simulink model "Microwave"  (Simulink 8.7)
settings: Solver=ode45  StartTime=0.0  StopTime=20  RelTol=1e-3
libraries: simulink x16
settings Model: Creator=bourbouh  LastModifiedBy=bourbouh
settings DataIOCC: SaveFormat=Structure
settings DebuggingCC: UnderspecifiedInitializationDetection=Simplified  MergeDetectMultiDrivingBlocksExec=error

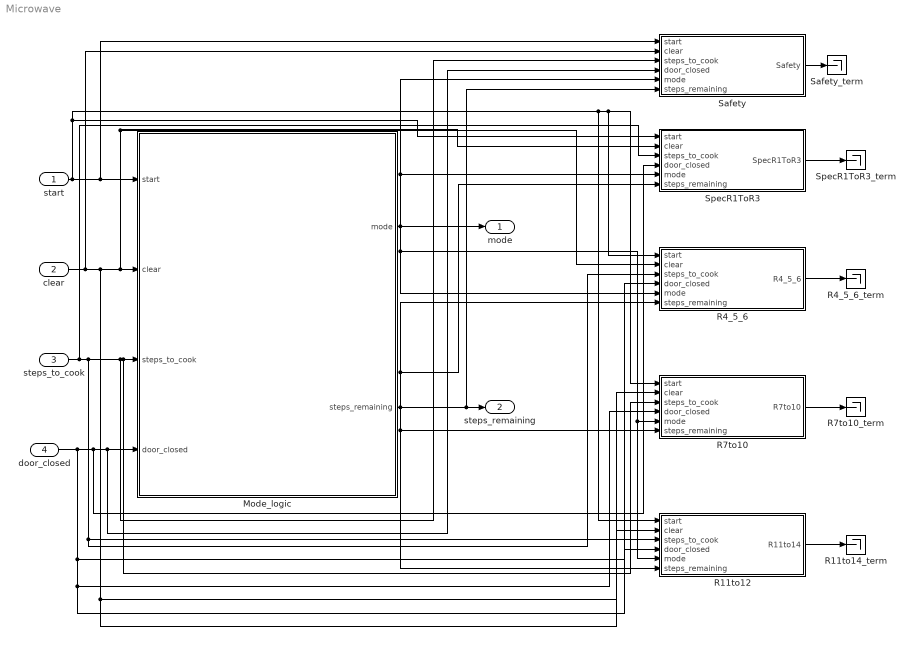
== system Microwave ==
  start : Inport
  clear : Inport  Port=2
  steps_to_cook : Inport  Port=3
  door_closed : Inport  Port=4
  Mode_logic : Stateflow chart  TreatAsAtomicUnit=on
  R11to12 : Subsystem  TreatAsAtomicUnit=on  mask(Observer){AnnotationType=ensures, ObserverType=[]}
      mask prompts: AnnotationType "Type of annotation (pre/post...)"; ObserverType "Observer type"
      mask help:
      | Set an observer for the system.
      | The annotation type parameter sets the type of observer:
      | - requires : pre-condition
      | - ensures : post-condition
      | - assert : an assertion
      | - observer : the observer computes a special type of properties
      mask TypeOptions AnnotationType: ensures | requires | assert | observer
      mask Callback AnnotationType:
      | paramStr = get_param(gcb, 'MaskValues');
      | if strcmp(paramStr{1}(1),'o')
      | set_param(gcb,'MaskVisibilities',{'on';'on'});
      | paramStr{2} = 'ellipsoid';
      | set_param(gcb,'MaskValues',paramStr);
      | else
      | set_param(gcb,'MaskVisibilities',{'on';'off'});
      | end
      | clear paramStr;
      mask Callback ObserverType:
      | paramStr = get_param(gcb, 'MaskValues');
      | if strcmp(paramStr{1}(1),'o')
      | set_param(gcb,'MaskVisibilities',{'on';'on'});
      | paramStr{2} = 'ellipsoid';
      | set_param(gcb,'MaskValues',paramStr);
      | else
      | set_param(gcb,'MaskVisibilities',{'on';'off'});
      | end
      | clear paramStr;
      mask Display:
      | color('black')
      | text(0.5, 0.5, ['Property: ''' get_param(gcb,'name') ''''], 'horizontalAlignment', 'center');
      | text(0.99, 0.03, '{\bf\fontsize{12}SAFE}', 'hor', 'right', 'ver', 'bottom', 'texmode', 'on');
  R11to14_term : Terminator
  R4_5_6 : Subsystem  TreatAsAtomicUnit=on  mask(Observer){AnnotationType=ensures, ObserverType=[]}
      mask prompts: AnnotationType "Type of annotation (pre/post...)"; ObserverType "Observer type"
      mask help:
      | Set an observer for the system.
      | The annotation type parameter sets the type of observer:
      | - requires : pre-condition
      | - ensures : post-condition
      | - assert : an assertion
      | - observer : the observer computes a special type of properties
      mask TypeOptions AnnotationType: ensures | requires | assert | observer
      mask Callback AnnotationType:
      | paramStr = get_param(gcb, 'MaskValues');
      | if strcmp(paramStr{1}(1),'o')
      | set_param(gcb,'MaskVisibilities',{'on';'on'});
      | paramStr{2} = 'ellipsoid';
      | set_param(gcb,'MaskValues',paramStr);
      | else
      | set_param(gcb,'MaskVisibilities',{'on';'off'});
      | end
      | clear paramStr;
      mask Callback ObserverType:
      | paramStr = get_param(gcb, 'MaskValues');
      | if strcmp(paramStr{1}(1),'o')
      | set_param(gcb,'MaskVisibilities',{'on';'on'});
      | paramStr{2} = 'ellipsoid';
      | set_param(gcb,'MaskValues',paramStr);
      | else
      | set_param(gcb,'MaskVisibilities',{'on';'off'});
      | end
      | clear paramStr;
      mask Display:
      | color('black')
      | text(0.5, 0.5, ['Property: ''' get_param(gcb,'name') ''''], 'horizontalAlignment', 'center');
      | text(0.99, 0.03, '{\bf\fontsize{12}SAFE}', 'hor', 'right', 'ver', 'bottom', 'texmode', 'on');
  R4_5_6_term : Terminator
  R7to10 : Subsystem  TreatAsAtomicUnit=on  mask(Observer){AnnotationType=ensures, ObserverType=[]}
      mask prompts: AnnotationType "Type of annotation (pre/post...)"; ObserverType "Observer type"
      mask help:
      | Set an observer for the system.
      | The annotation type parameter sets the type of observer:
      | - requires : pre-condition
      | - ensures : post-condition
      | - assert : an assertion
      | - observer : the observer computes a special type of properties
      mask TypeOptions AnnotationType: ensures | requires | assert | observer
      mask Callback AnnotationType:
      | paramStr = get_param(gcb, 'MaskValues');
      | if strcmp(paramStr{1}(1),'o')
      | set_param(gcb,'MaskVisibilities',{'on';'on'});
      | paramStr{2} = 'ellipsoid';
      | set_param(gcb,'MaskValues',paramStr);
      | else
      | set_param(gcb,'MaskVisibilities',{'on';'off'});
      | end
      | clear paramStr;
      mask Callback ObserverType:
      | paramStr = get_param(gcb, 'MaskValues');
      | if strcmp(paramStr{1}(1),'o')
      | set_param(gcb,'MaskVisibilities',{'on';'on'});
      | paramStr{2} = 'ellipsoid';
      | set_param(gcb,'MaskValues',paramStr);
      | else
      | set_param(gcb,'MaskVisibilities',{'on';'off'});
      | end
      | clear paramStr;
      mask Display:
      | color('black')
      | text(0.5, 0.5, ['Property: ''' get_param(gcb,'name') ''''], 'horizontalAlignment', 'center');
      | text(0.99, 0.03, '{\bf\fontsize{12}SAFE}', 'hor', 'right', 'ver', 'bottom', 'texmode', 'on');
  R7to10_term : Terminator
  Safety : Subsystem  TreatAsAtomicUnit=on  mask(Observer){AnnotationType=ensures, ObserverType=[]}
      mask prompts: AnnotationType "Type of annotation (pre/post...)"; ObserverType "Observer type"
      mask help:
      | Set an observer for the system.
      | The annotation type parameter sets the type of observer:
      | - requires : pre-condition
      | - ensures : post-condition
      | - assert : an assertion
      | - observer : the observer computes a special type of properties
      mask TypeOptions AnnotationType: ensures | requires | assert | observer
      mask Callback AnnotationType:
      | paramStr = get_param(gcb, 'MaskValues');
      | if strcmp(paramStr{1}(1),'o')
      | set_param(gcb,'MaskVisibilities',{'on';'on'});
      | paramStr{2} = 'ellipsoid';
      | set_param(gcb,'MaskValues',paramStr);
      | else
      | set_param(gcb,'MaskVisibilities',{'on';'off'});
      | end
      | clear paramStr;
      mask Callback ObserverType:
      | paramStr = get_param(gcb, 'MaskValues');
      | if strcmp(paramStr{1}(1),'o')
      | set_param(gcb,'MaskVisibilities',{'on';'on'});
      | paramStr{2} = 'ellipsoid';
      | set_param(gcb,'MaskValues',paramStr);
      | else
      | set_param(gcb,'MaskVisibilities',{'on';'off'});
      | end
      | clear paramStr;
      mask Display:
      | color('black')
      | text(0.5, 0.5, ['Property: ''' get_param(gcb,'name') ''''], 'horizontalAlignment', 'center');
      | text(0.99, 0.03, '{\bf\fontsize{12}SAFE}', 'hor', 'right', 'ver', 'bottom', 'texmode', 'on');
  Safety_term : Terminator
  SpecR1ToR3 : Subsystem  TreatAsAtomicUnit=on  mask(Observer){AnnotationType=ensures, ObserverType=[]}
      mask prompts: AnnotationType "Type of annotation (pre/post...)"; ObserverType "Observer type"
      mask help:
      | Set an observer for the system.
      | The annotation type parameter sets the type of observer:
      | - requires : pre-condition
      | - ensures : post-condition
      | - assert : an assertion
      | - observer : the observer computes a special type of properties
      mask TypeOptions AnnotationType: ensures | requires | assert | observer
      mask Callback AnnotationType:
      | paramStr = get_param(gcb, 'MaskValues');
      | if strcmp(paramStr{1}(1),'o')
      | set_param(gcb,'MaskVisibilities',{'on';'on'});
      | paramStr{2} = 'ellipsoid';
      | set_param(gcb,'MaskValues',paramStr);
      | else
      | set_param(gcb,'MaskVisibilities',{'on';'off'});
      | end
      | clear paramStr;
      mask Callback ObserverType:
      | paramStr = get_param(gcb, 'MaskValues');
      | if strcmp(paramStr{1}(1),'o')
      | set_param(gcb,'MaskVisibilities',{'on';'on'});
      | paramStr{2} = 'ellipsoid';
      | set_param(gcb,'MaskValues',paramStr);
      | else
      | set_param(gcb,'MaskVisibilities',{'on';'off'});
      | end
      | clear paramStr;
      mask Display:
      | color('black')
      | text(0.5, 0.5, ['Property: ''' get_param(gcb,'name') ''''], 'horizontalAlignment', 'center');
      | text(0.99, 0.03, '{\bf\fontsize{12}SAFE}', 'hor', 'right', 'ver', 'bottom', 'texmode', 'on');
  SpecR1ToR3_term : Terminator
  mode : Outport
  steps_remaining : Outport  Port=2
  wires:
  start/1 -> R11to12/1(start), R7to10/1(start), R4_5_6/1(start), SpecR1ToR3/1(start), Safety/1(start), Mode_logic/1(start)
  door_closed/1 -> R11to12/4(door_closed), R7to10/4(door_closed), R4_5_6/4(door_closed), Mode_logic/4(door_closed), Safety/4(door_closed), SpecR1ToR3/4(door_closed)
  steps_to_cook/1 -> R11to12/3(steps_to_cook), R4_5_6/3(steps_to_cook), R7to10/3(steps_to_cook), Mode_logic/3(steps_to_cook), Safety/3(steps_to_cook), SpecR1ToR3/3(steps_to_cook)
  clear/1 -> R11to12/2(clear), R7to10/2(clear), R4_5_6/2(clear), SpecR1ToR3/2(clear), Mode_logic/2(clear), Safety/2(clear)
  Mode_logic/1(mode) -> R11to12/5(mode), R7to10/5(mode), R4_5_6/5(mode), Safety/5(mode), SpecR1ToR3/5(mode), mode/1
  Mode_logic/2(steps_remaining) -> R7to10/6(steps_remaining), R11to12/6(steps_remaining), SpecR1ToR3/6(steps_remaining), R4_5_6/6(steps_remaining), steps_remaining/1, Safety/6(steps_remaining)
  Safety/1(Safety) -> Safety_term/1
  SpecR1ToR3/1(SpecR1ToR3) -> SpecR1ToR3_term/1
  R4_5_6/1(R4_5_6) -> R4_5_6_term/1
  R7to10/1(R7to10) -> R7to10_term/1
  R11to12/1(R11to14) -> R11to14_term/1

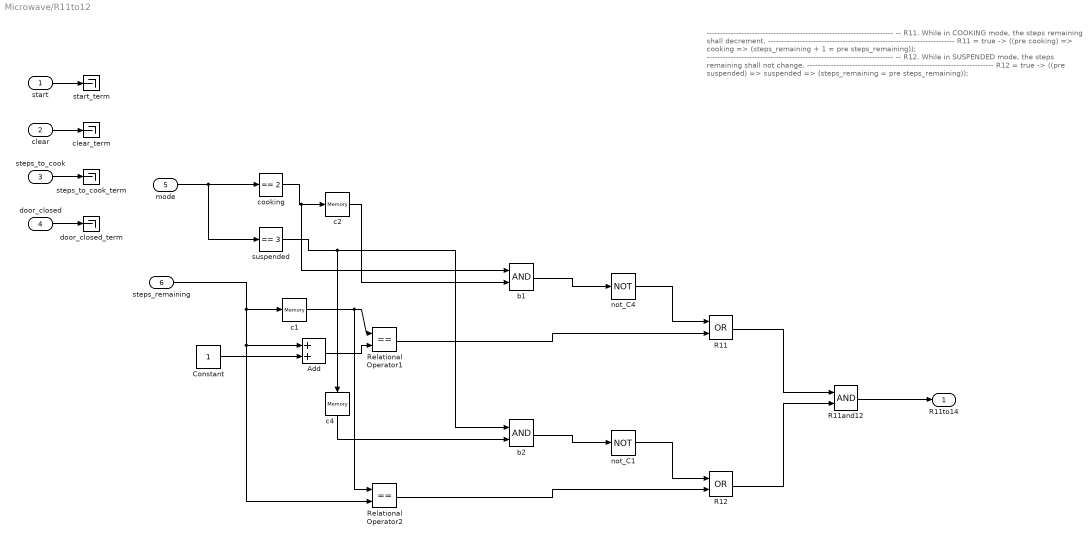
== system Microwave/R11to12 ==
  note: ----------------------------------------------------------------------
      | -- R11. While in COOKING mode, the steps remaining shall decrement.
      | ----------------------------------------------------------------------
      | R11 = true -> ((pre cooking) => cooking => (steps_remaining + 1 = pre steps_remaining));
      |
      | ----------------------------------------------------------------------
      | -- R12. While in SUSPENDED mode, the steps remaining shall not change.
      | ----------------------------------------------------------------------
      | R12 = true -> ((pre suspended) => suspended => (steps_remaining = pre steps_remaining));
  start : Inport
  clear : Inport  Port=2
  steps_to_cook : Inport  Port=3
  door_closed : Inport  Port=4
  mode : Inport  Port=5
  steps_remaining : Inport  Port=6
  Add : Sum
  Constant : Constant  OutDataTypeStr=int32
  R11 : Logic  Operator=OR  AllPortsSameDT=off  OutDataTypeStr=boolean
  R11and12 : Logic  AllPortsSameDT=off  OutDataTypeStr=boolean
  R12 : Logic  Operator=OR  AllPortsSameDT=off  OutDataTypeStr=boolean
  Relational Operator1 : RelationalOperator  Operator===  OutDataTypeStr=boolean
  Relational Operator2 : RelationalOperator  Operator===  OutDataTypeStr=boolean
  b1 : Logic  AllPortsSameDT=off  OutDataTypeStr=boolean
  b2 : Logic  AllPortsSameDT=off  OutDataTypeStr=boolean
  c1 : Memory  X0=false
  c2 : Memory  X0=false
  c4 : Memory  X0=false
  clear_term : Terminator
  cooking : simulink/Logic and Bit Operations/Compare To Constant  relop===  const=2  OutDataTypeStr=boolean
  door_closed_term : Terminator
  not_C1 : Logic  Operator=NOT  AllPortsSameDT=off  OutDataTypeStr=boolean
  not_C4 : Logic  Operator=NOT  AllPortsSameDT=off  OutDataTypeStr=boolean
  start_term : Terminator
  steps_to_cook_term : Terminator
  suspended : simulink/Logic and Bit Operations/Compare To Constant  relop===  const=3  OutDataTypeStr=boolean
  R11to14 : Outport
  wires:
  start/1 -> start_term/1
  clear/1 -> clear_term/1
  steps_to_cook/1 -> steps_to_cook_term/1
  door_closed/1 -> door_closed_term/1
  cooking/1 -> c2/1, b1/1
  c2/1 -> b1/2
  Add/1 -> Relational Operator1/2
  b1/1 -> not_C4/1
  not_C4/1 -> R11/1
  Relational Operator1/1 -> R11/2
  R11/1 -> R11and12/1
  mode/1 -> cooking/1, suspended/1
  Constant/1 -> Add/2
  suspended/1 -> b2/1, c4/1
  c1/1 -> Relational Operator2/1, Relational Operator1/1
  b2/1 -> not_C1/1
  not_C1/1 -> R12/1
  Relational Operator2/1 -> R12/2
  R12/1 -> R11and12/2
  steps_remaining/1 -> Relational Operator2/2, Add/1, c1/1
  c4/1 -> b2/2
  R11and12/1 -> R11to14/1

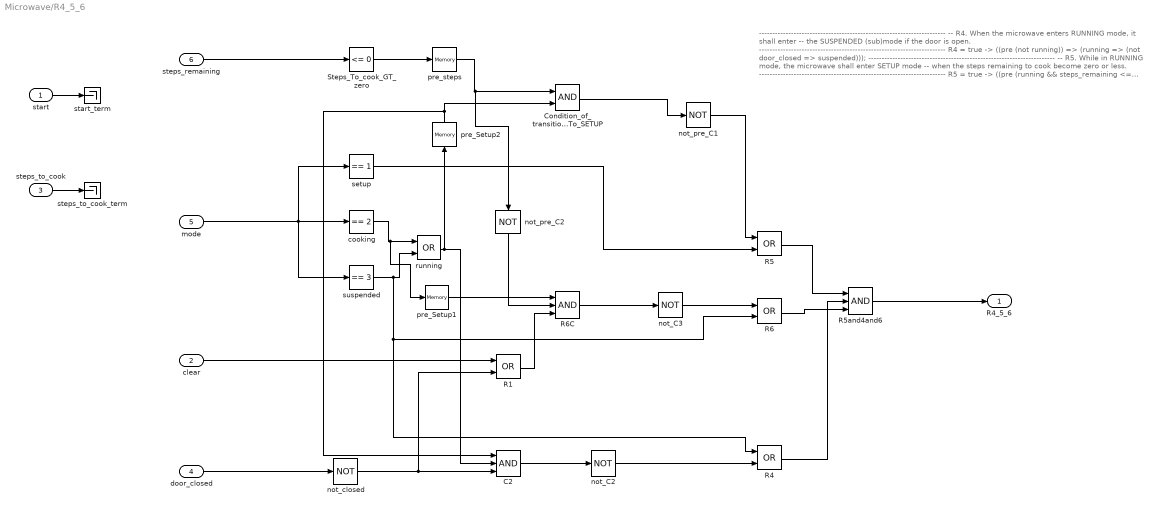
== system Microwave/R4_5_6 ==
  note: ----------------------------------------------------------------------
      | -- R4. When the microwave enters RUNNING mode, it shall enter
      | -- the SUSPENDED (sub)mode if the door is open.
      | ----------------------------------------------------------------------
      | R4 = true -> ((pre (not running)) => (running => (not door_closed => suspended)));
      |
      | ----------------------------------------------------------------------
      | -- R5. While in RUNNING mode, the microwave shall enter SETUP mode
      | -- when the steps remaining to cook become zero or less.
      | ----------------------------------------------------------------------
      | R5 = true -> ((pre (running && steps_remaining <= 0)) => setup);
      |
      | ----------------------------------------------------------------------
      | -- R6. While in COOKING mode, the microwave shall enter SUSPENDED
      | -- mode if the door is opened or the clear key is pressed.
      | ----------------------------------------------------------------------
      | R6 = true -> ((pre (cooking && steps_remaining > 0)) =>
      | (not door_closed || clear) => suspended);
  start : Inport
  clear : Inport  Port=2
  steps_to_cook : Inport  Port=3
  door_closed : Inport  Port=4
  mode : Inport  Port=5
  steps_remaining : Inport  Port=6
  C2 : Logic  Inputs=3  AllPortsSameDT=off  OutDataTypeStr=boolean
  Condition_of_transition_RUNNING_To_SETUP : Logic  AllPortsSameDT=off  OutDataTypeStr=boolean
  R{1,4..6} (4 alike) : Logic  Operator=OR  AllPortsSameDT=off  OutDataTypeStr=boolean
  R5and4and6 : Logic  Inputs=3  AllPortsSameDT=off  OutDataTypeStr=boolean
  R6C : Logic  Inputs=3  AllPortsSameDT=off  OutDataTypeStr=boolean
  Steps_To_cook_GT_zero : simulink/Logic and Bit Operations/Compare To Constant  relop=<=  const=0  OutDataTypeStr=boolean
  cooking : simulink/Logic and Bit Operations/Compare To Constant  relop===  const=2  OutDataTypeStr=boolean
  not_C2 : Logic  Operator=NOT  AllPortsSameDT=off  OutDataTypeStr=boolean
  not_C3 : Logic  Operator=NOT  AllPortsSameDT=off  OutDataTypeStr=boolean
  not_closed : Logic  Operator=NOT  AllPortsSameDT=off  OutDataTypeStr=boolean
  not_pre_C1 : Logic  Operator=NOT  AllPortsSameDT=off  OutDataTypeStr=boolean
  not_pre_C2 : Logic  Operator=NOT  AllPortsSameDT=off  OutDataTypeStr=boolean
  pre_Setup1 : Memory  X0=false
  pre_Setup2 : Memory  X0=false
  pre_steps : Memory  X0=false
  running : Logic  Operator=OR  AllPortsSameDT=off  OutDataTypeStr=boolean
  setup : simulink/Logic and Bit Operations/Compare To Constant  relop===  const=1  OutDataTypeStr=boolean
  start_term : Terminator
  steps_to_cook_term : Terminator
  suspended : simulink/Logic and Bit Operations/Compare To Constant  relop===  const=3  OutDataTypeStr=boolean
  R4_5_6 : Outport
  wires:
  start/1 -> start_term/1
  clear/1 -> R1/1
  steps_to_cook/1 -> steps_to_cook_term/1
  door_closed/1 -> not_closed/1
  suspended/1 -> R4/1, R6/2, running/2
  running/1 -> C2/2, pre_Setup2/1
  not_pre_C1/1 -> R5/1
  R5/1 -> R5and4and6/1
  Condition_of_transition_RUNNING_To_SETUP/1 -> not_pre_C1/1
  Steps_To_cook_GT_zero/1 -> pre_steps/1
  not_C2/1 -> R4/2
  cooking/1 -> pre_Setup1/1, running/1
  R4/1 -> R5and4and6/2
  mode/1 -> suspended/1, setup/1, cooking/1
  pre_Setup2/1 -> Condition_of_transition_RUNNING_To_SETUP/2, C2/1
  C2/1 -> not_C2/1
  not_closed/1 -> R1/2, C2/3
  steps_remaining/1 -> Steps_To_cook_GT_zero/1
  pre_steps/1 -> Condition_of_transition_RUNNING_To_SETUP/1, not_pre_C2/1
  setup/1 -> R5/2
  pre_Setup1/1 -> R6C/1
  not_pre_C2/1 -> R6C/2
  R1/1 -> R6C/3
  R6C/1 -> not_C3/1
  not_C3/1 -> R6/1
  R6/1 -> R5and4and6/3
  R5and4and6/1 -> R4_5_6/1

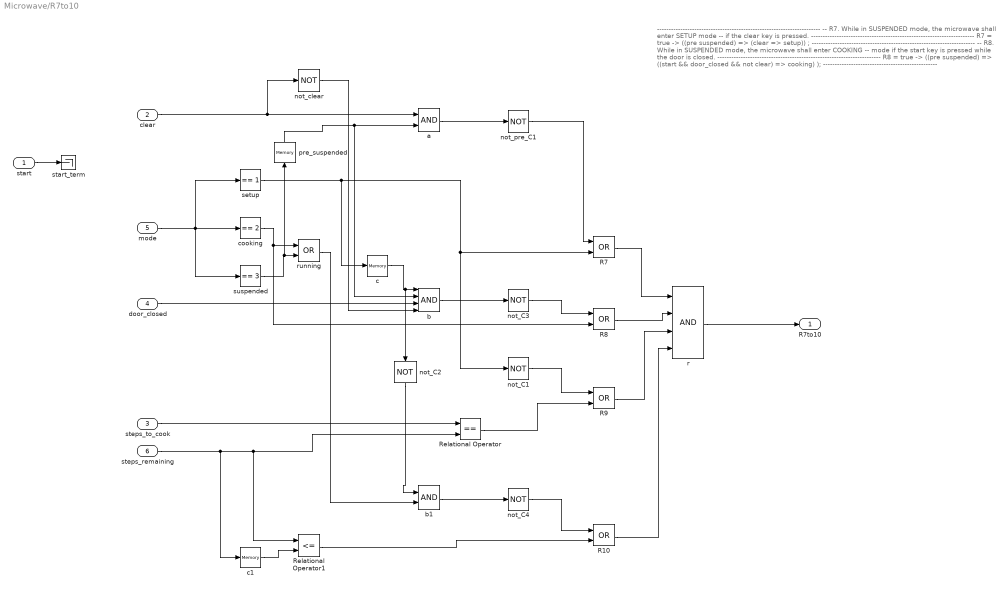
== system Microwave/R7to10 ==
  note: ----------------------------------------------------------------------
      | -- R7. While in SUSPENDED mode, the microwave shall enter SETUP mode
      | -- if the clear key is pressed.
      | ----------------------------------------------------------------------
      | R7 = true -> ((pre suspended) => (clear => setup)) ;
      |
      | ----------------------------------------------------------------------
      | -- R8. While in SUSPENDED mode, the microwave shall enter COOKING
      | -- mode if the start key is pressed while the door is closed.
      | ----------------------------------------------------------------------
      | R8 = true -> ((pre suspended) => ((start && door_closed && not clear) => cooking) );
      |
      | ----------------------------------------------------------------------
      | -- R9. While in SETUP mode, the steps remaining to cook shall be
      | -- set to the steps to cook (to ensure the display agrees with the
      | -- time the user has entered so far).
      | ----------------------------------------------------------------------
      | R9 = setup => steps_remaining = steps_to_cook;
      |
      | ----------------------------------------------------------------------
      | -- R10. While in RUNNING mode, the steps remaining shall never
      | -- increase.
      | ----------------------------------------------------------------------
      | R10 = true -> ((pre running) => running => (steps_remaining <= pre steps_remaining));
  start : Inport
  clear : Inport  Port=2
  steps_to_cook : Inport  Port=3
  door_closed : Inport  Port=4
  mode : Inport  Port=5
  steps_remaining : Inport  Port=6
  R{7..10} (4 alike) : Logic  Operator=OR  AllPortsSameDT=off  OutDataTypeStr=boolean
  Relational Operator : RelationalOperator  Operator===  OutDataTypeStr=boolean
  Relational Operator1 : RelationalOperator  Operator=<=  OutDataTypeStr=boolean
  a : Logic  AllPortsSameDT=off  OutDataTypeStr=boolean
  b : Logic  Inputs=4  AllPortsSameDT=off  OutDataTypeStr=boolean
  b1 : Logic  AllPortsSameDT=off  OutDataTypeStr=boolean
  c : Memory  X0=false
  c1 : Memory  X0=false
  cooking : simulink/Logic and Bit Operations/Compare To Constant  relop===  const=2  OutDataTypeStr=boolean
  not_C{1..4} (4 alike) : Logic  Operator=NOT  AllPortsSameDT=off  OutDataTypeStr=boolean
  not_clear : Logic  Operator=NOT  AllPortsSameDT=off  OutDataTypeStr=boolean
  not_pre_C1 : Logic  Operator=NOT  AllPortsSameDT=off  OutDataTypeStr=boolean
  pre_suspended : Memory  X0=false
  r : Logic  Inputs=4  AllPortsSameDT=off  OutDataTypeStr=boolean
  running : Logic  Operator=OR  AllPortsSameDT=off  OutDataTypeStr=boolean
  setup : simulink/Logic and Bit Operations/Compare To Constant  relop===  const=1  OutDataTypeStr=boolean
  start_term : Terminator
  suspended : simulink/Logic and Bit Operations/Compare To Constant  relop===  const=3  OutDataTypeStr=boolean
  R7to10 : Outport
  wires:
  start/1 -> start_term/1
  steps_to_cook/1 -> Relational Operator/1
  door_closed/1 -> b/3
  steps_remaining/1 -> c1/1, Relational Operator1/1, Relational Operator/2
  suspended/1 -> pre_suspended/1, running/2
  not_pre_C1/1 -> R7/1
  R7/1 -> r/1
  a/1 -> not_pre_C1/1
  cooking/1 -> running/1, R8/2
  mode/1 -> suspended/1, setup/1, cooking/1
  setup/1 -> c/1, not_C1/1, R7/2
  c/1 -> not_C2/1, b/1
  pre_suspended/1 -> b/2, a/2
  b/1 -> not_C3/1
  not_C3/1 -> R8/1
  R8/1 -> r/2
  clear/1 -> not_clear/1, a/1
  not_clear/1 -> b/4
  not_C1/1 -> R9/1
  Relational Operator/1 -> R9/2
  R9/1 -> r/3
  not_C2/1 -> b1/1
  running/1 -> b1/2
  c1/1 -> Relational Operator1/2
  b1/1 -> not_C4/1
  not_C4/1 -> R10/1
  Relational Operator1/1 -> R10/2
  R10/1 -> r/4
  r/1 -> R7to10/1

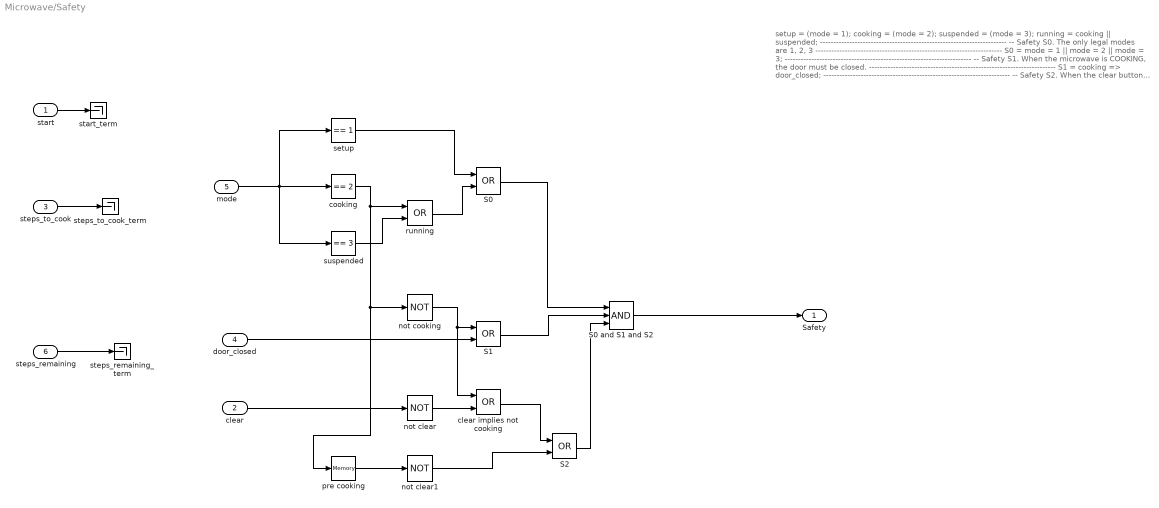
== system Microwave/Safety ==
  note: setup = (mode = 1);
      | cooking = (mode = 2);
      | suspended = (mode = 3);
      | running = cooking || suspended;
      |
      | ----------------------------------------------------------------------
      | -- Safety S0. The only legal modes are 1, 2, 3
      | ----------------------------------------------------------------------
      | S0 = mode = 1 || mode = 2 || mode = 3;
      |
      | ----------------------------------------------------------------------
      | -- Safety S1. When the microwave is COOKING, the door must be closed.
      | ----------------------------------------------------------------------
      | S1 = cooking => door_closed;
      |
      | ----------------------------------------------------------------------
      | -- Safety S2. When the clear button is pressed, the microwave will
      | -- stop cooking.
      | ----------------------------------------------------------------------
      | S2 = true -> ((pre cooking) => (clear => not cooking));
  start : Inport
  clear : Inport  Port=2
  steps_to_cook : Inport  Port=3
  door_closed : Inport  Port=4
  mode : Inport  Port=5
  steps_remaining : Inport  Port=6
  S0 : Logic  Operator=OR  AllPortsSameDT=off  OutDataTypeStr=boolean
  S0 and S1 and S2 : Logic  Inputs=3  AllPortsSameDT=off  OutDataTypeStr=boolean
  S1 : Logic  Operator=OR  AllPortsSameDT=off  OutDataTypeStr=boolean
  S2 : Logic  Operator=OR  AllPortsSameDT=off  OutDataTypeStr=boolean
  clear implies not cooking : Logic  Operator=OR  AllPortsSameDT=off  OutDataTypeStr=boolean
  cooking : simulink/Logic and Bit Operations/Compare To Constant  relop===  const=2  OutDataTypeStr=boolean
  not clear : Logic  Operator=NOT  AllPortsSameDT=off  OutDataTypeStr=boolean
  not clear1 : Logic  Operator=NOT  AllPortsSameDT=off  OutDataTypeStr=boolean
  not cooking : Logic  Operator=NOT  AllPortsSameDT=off  OutDataTypeStr=boolean
  pre cooking : Memory
  running : Logic  Operator=OR  AllPortsSameDT=off  OutDataTypeStr=boolean
  setup : simulink/Logic and Bit Operations/Compare To Constant  relop===  const=1  OutDataTypeStr=boolean
  start_term : Terminator
  steps_remaining_term : Terminator
  steps_to_cook_term : Terminator
  suspended : simulink/Logic and Bit Operations/Compare To Constant  relop===  const=3  OutDataTypeStr=boolean
  Safety : Outport
  wires:
  start/1 -> start_term/1
  clear/1 -> not clear/1
  steps_to_cook/1 -> steps_to_cook_term/1
  door_closed/1 -> S1/2
  mode/1 -> suspended/1, setup/1, cooking/1
  steps_remaining/1 -> steps_remaining_term/1
  cooking/1 -> running/1, not cooking/1, pre cooking/1
  suspended/1 -> running/2
  setup/1 -> S0/1
  running/1 -> S0/2
  not cooking/1 -> clear implies not cooking/1, S1/1
  S0/1 -> S0 and S1 and S2/1
  S1/1 -> S0 and S1 and S2/2
  not clear/1 -> clear implies not cooking/2
  clear implies not cooking/1 -> S2/1
  pre cooking/1 -> not clear1/1
  not clear1/1 -> S2/2
  S2/1 -> S0 and S1 and S2/3
  S0 and S1 and S2/1 -> Safety/1

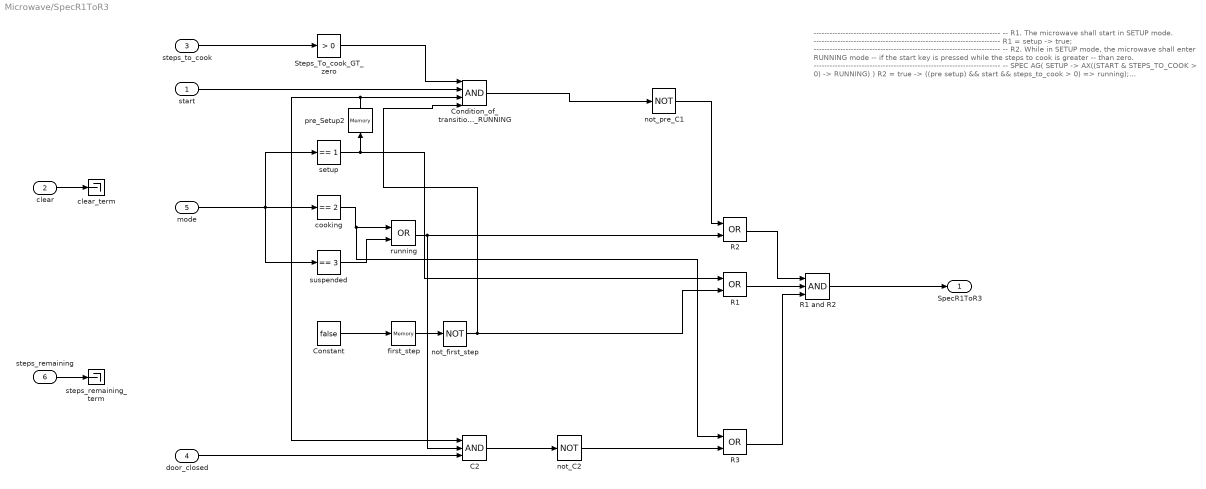
== system Microwave/SpecR1ToR3 ==
  note: ----------------------------------------------------------------------
      | -- R1. The microwave shall start in SETUP mode.
      | ----------------------------------------------------------------------
      | R1 = setup -> true;
      |
      | ----------------------------------------------------------------------
      | -- R2. While in SETUP mode, the microwave shall enter RUNNING mode
      | -- if the start key is pressed while the steps to cook is greater
      | -- than zero.
      | ----------------------------------------------------------------------
      | -- SPEC AG( SETUP -> AX((START & STEPS_TO_COOK > 0) -> RUNNING) )
      |
      | R2 = true -> ((pre setup) && start && steps_to_cook > 0) => running);
      |
      | ----------------------------------------------------------------------
      | -- R3. When the microwave enters RUNNING mode, it shall enter
      | -- the COOKING (sub)mode if the door is closed.
      | ----------------------------------------------------------------------
      | R3 = true -> ((pre (not running)) => (running => (door_closed => cooking)));
  start : Inport
  clear : Inport  Port=2
  steps_to_cook : Inport  Port=3
  door_closed : Inport  Port=4
  mode : Inport  Port=5
  steps_remaining : Inport  Port=6
  C2 : Logic  Inputs=3  AllPortsSameDT=off  OutDataTypeStr=boolean
  Condition_of_transition_SETUP_To_RUNNING : Logic  Inputs=4  AllPortsSameDT=off  OutDataTypeStr=boolean
  Constant : Constant  Value=false  OutDataTypeStr=boolean
  R1 : Logic  Operator=OR  AllPortsSameDT=off  OutDataTypeStr=boolean
  R1 and R2 : Logic  Inputs=3  AllPortsSameDT=off  OutDataTypeStr=boolean
  R2 : Logic  Operator=OR  AllPortsSameDT=off  OutDataTypeStr=boolean
  R3 : Logic  Operator=OR  AllPortsSameDT=off  OutDataTypeStr=boolean
  Steps_To_cook_GT_zero : simulink/Logic and Bit Operations/Compare To Constant  relop=>  const=0  OutDataTypeStr=boolean
  clear_term : Terminator
  cooking : simulink/Logic and Bit Operations/Compare To Constant  relop===  const=2  OutDataTypeStr=boolean
  first_step : Memory  X0=true
  not_C2 : Logic  Operator=NOT  AllPortsSameDT=off  OutDataTypeStr=boolean
  not_first_step : Logic  Operator=NOT  AllPortsSameDT=off  OutDataTypeStr=boolean
  not_pre_C1 : Logic  Operator=NOT  AllPortsSameDT=off  OutDataTypeStr=boolean
  pre_Setup2 : Memory  X0=false
  running : Logic  Operator=OR  AllPortsSameDT=off  OutDataTypeStr=boolean
  setup : simulink/Logic and Bit Operations/Compare To Constant  relop===  const=1  OutDataTypeStr=boolean
  steps_remaining_term : Terminator
  suspended : simulink/Logic and Bit Operations/Compare To Constant  relop===  const=3  OutDataTypeStr=boolean
  SpecR1ToR3 : Outport
  wires:
  clear/1 -> clear_term/1
  door_closed/1 -> C2/3
  steps_remaining/1 -> steps_remaining_term/1
  suspended/1 -> running/2
  Constant/1 -> first_step/1
  first_step/1 -> not_first_step/1
  not_first_step/1 -> R1/2, Condition_of_transition_SETUP_To_RUNNING/4
  running/1 -> R2/2, C2/2
  not_pre_C1/1 -> R2/1
  R1/1 -> R1 and R2/2
  R2/1 -> R1 and R2/1
  setup/1 -> pre_Setup2/1, R1/1
  steps_to_cook/1 -> Steps_To_cook_GT_zero/1
  Condition_of_transition_SETUP_To_RUNNING/1 -> not_pre_C1/1
  start/1 -> Condition_of_transition_SETUP_To_RUNNING/2
  Steps_To_cook_GT_zero/1 -> Condition_of_transition_SETUP_To_RUNNING/1
  not_C2/1 -> R3/2
  cooking/1 -> R3/1, running/1
  R3/1 -> R1 and R2/3
  mode/1 -> suspended/1, setup/1, cooking/1
  pre_Setup2/1 -> Condition_of_transition_SETUP_To_RUNNING/3, C2/1
  C2/1 -> not_C2/1
  R1 and R2/1 -> SpecR1ToR3/1

== stateflow chart Mode_logic ==
  settings: updateMethod=DISCRETE  sampleTime=1
  state SETUP
    entry:
    mode=1;
    steps_remaining = steps_to_cook;
  state RUNNING
    state COOKING
      entry: mode=2;
    state SUSPENDED
      entry: mode=3;
    COOKING -> COOKING [order 2] : [steps_remaining > 0]
        | /steps_remaining--;
    (default) -> (junction 7)
    (junction 7) -> COOKING [order 1] : [door_closed]
    (junction 7) -> SUSPENDED [order 2]
    SUSPENDED -> COOKING [order 2] : [start && ...
        | door_closed]
    COOKING -> SUSPENDED [order 1] : [clear || ...
        | !door_closed]
  (default) -> SETUP
  SETUP -> (junction 20) : {steps_remaining = steps_to_cook;}
  (junction 20) -> RUNNING : [start && steps_remaining > 0]
  (junction 21) -> SETUP
  RUNNING -> (junction 21) : [steps_remaining <= 0]
  SUSPENDED -> (junction 21) [order 1] : [clear]
  data: start input boolean; clear input boolean; steps_to_cook input uint16; door_closed input boolean; mode output uint8; steps_remaining output uint16 [0..600]
